simulink model "Vehicle3DOFModelwithLonnLatController"  (R2019b)
settings: Solver=FixedStepAuto  StartTime=0.0  StopTime=150  FixedStep=0.05  RelTol=1e-3
values from neighbouring files (symbols this model uses):
  Ks = 0.1    [Vehicle_Parameters_and_initial_state_comp.m]
  Kv = -10    [Vehicle_Parameters_and_initial_state_comp.m]    (also in sfun_LQRwithFF_YC_2DOF_Vx_changed.m = m/2/L*(lr/Kyf-lf/Kyr))
  m = car.m    [Vehicle_Parameters_and_initial_state_comp.m]    (also in sfun_LQRwithFF_YC_2DOF_Vx_changed.m)
  t_end = 44    [Vehicle_Parameters_and_initial_state_comp.m]
  Ta = 0.1    [Vehicle_Parameters_and_initial_state_comp.m]
  VehPar = [g,m,Iz,lf,lr,l,Kyf,Kyr,mu,FzF,FzR,FxR_max]'    [Vehicle_Parameters_and_initial_state_comp.m]
  VehPos0 = [Tra(1,1);Tra(1,2);Tra(1,3)]    [Vehicle_Parameters_and_initial_state_comp.m]
  VehSt0 = [0;0;Tra(1,6)]    [Vehicle_Parameters_and_initial_state_comp.m]
undefined symbols (not defined in the file or in its folder): Tra
libraries: simulink x2
settings Model: Creator=pc  LastModifiedBy=YC

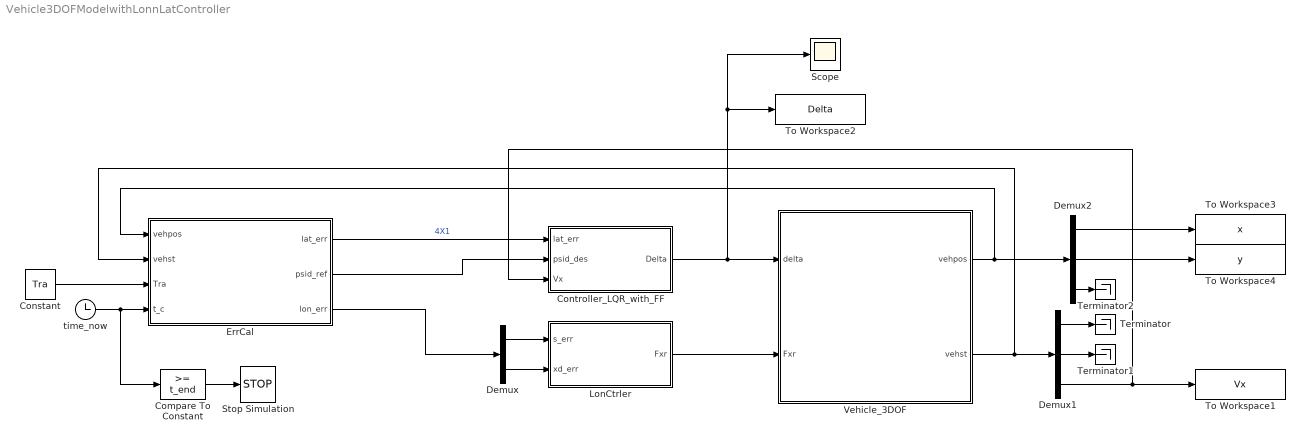
== system Vehicle3DOFModelwithLonnLatController ==
  Compare To Constant : simulink/Logic and Bit Operations/Compare To Constant  relop=>=  const=t_end  OutDataTypeStr=boolean
  Constant : Constant  Value=Tra
  Controller_LQR_with_FF : Subsystem  VariantControl=Controller_mode==1
  Demux : Demux  Outputs=2
  Demux1 : Demux  Outputs=3
  Demux2 : Demux  Outputs=3
  ErrCal : Subsystem  Variant=on
  LonCtrler : Subsystem
  Scope : Scope
  Stop Simulation : Stop
  Terminator : Terminator
  Terminator1 : Terminator
  Terminator2 : Terminator
  To Workspace1 : ToWorkspace  VariableName=Vx  SampleTime=-1
  To Workspace2 : ToWorkspace  VariableName=Delta  SampleTime=-1
  To Workspace3 : ToWorkspace  VariableName=x  SampleTime=-1
  To Workspace4 : ToWorkspace  VariableName=y  SampleTime=-1
  Vehicle_3DOF : Subsystem
  time_now : Clock
  wires:
  Controller_LQR_with_FF/1(Delta) -> To Workspace2/1, Scope/1, Vehicle_3DOF/1(delta)
  ErrCal/1(lat_err) -> Controller_LQR_with_FF/1(lat_err)  "4X1"
  ErrCal/2(psid_ref) -> Controller_LQR_with_FF/2(psid_des)
  LonCtrler/1(Fxr) -> Vehicle_3DOF/2(Fxr)
  Demux/1 -> LonCtrler/1(s_err)
  Demux/2 -> LonCtrler/2(xd_err)
  ErrCal/3(lon_err) -> Demux/1
  Vehicle_3DOF/1(vehpos) -> ErrCal/1(vehpos), Demux2/1
  Vehicle_3DOF/2(vehst) -> ErrCal/2(vehst), Demux1/1
  Constant/1 -> ErrCal/3(Tra)
  time_now/1 -> ErrCal/4(t_c), Compare To Constant/1
  Demux1/1 -> Terminator/1
  Demux1/2 -> Terminator1/1
  Demux1/3 -> To Workspace1/1, Controller_LQR_with_FF/3(Vx)
  Compare To Constant/1 -> Stop Simulation/1
  Demux2/3 -> Terminator2/1
  Demux2/2 -> To Workspace4/1
  Demux2/1 -> To Workspace3/1

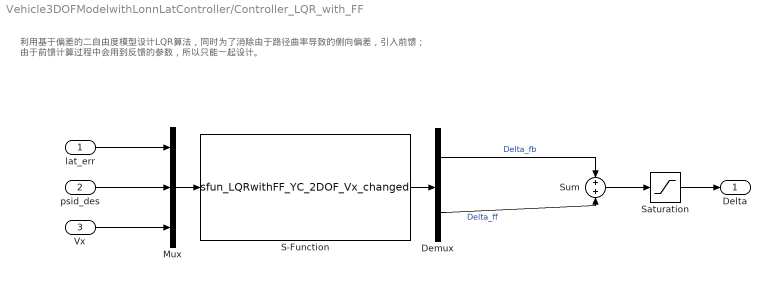
== system Vehicle3DOFModelwithLonnLatController/Controller_LQR_with_FF ==
  note: 利用基于偏差的二自由度模型设计LQR算法，同时为了消除由于路径曲率导致的侧向偏差，引入前馈；
      | 由于前馈计算过程中会用到反馈的参数，所以只能一起设计。
  lat_err : Inport
  psid_des : Inport  Port=2
  Vx : Inport  Port=3
  Demux : Demux  Outputs=2
  Mux : Mux  Inputs=3
  S-Function : S-Function  FunctionName=sfun_LQRwithFF_YC_2DOF_Vx_changed  Parameters=car  SFunctionDeploymentMode=off  EnableBusSupport=off
  Saturation : Saturate  UpperLimit=0.61  LowerLimit=-0.61
  Sum : Sum  Inputs=+|+
  Delta : Outport
  wires:
  Mux/1 -> S-Function/1
  Demux/2 -> Sum/2  "Delta_ff"
  Demux/1 -> Sum/1  "Delta_fb"
  Sum/1 -> Saturation/1
  S-Function/1 -> Demux/1
  lat_err/1 -> Mux/1
  psid_des/1 -> Mux/2
  Vx/1 -> Mux/3
  Saturation/1 -> Delta/1

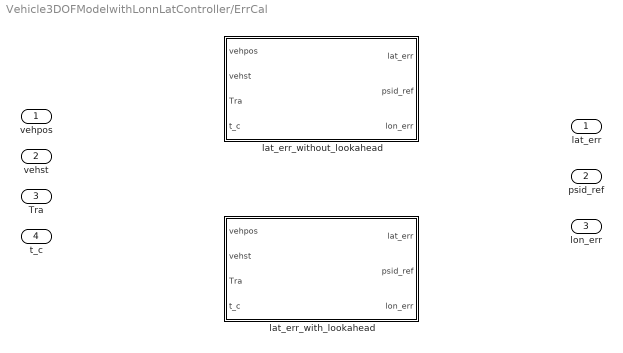
== system Vehicle3DOFModelwithLonnLatController/ErrCal ==
  vehpos : Inport
  vehst : Inport  Port=2
  Tra : Inport  Port=3
  t_c : Inport  Port=4
  lat_err_with_lookahead : Subsystem  VariantControl=Error_Mode==1
  lat_err_without_lookahead : Subsystem  VariantControl=Error_Mode==0
  lat_err : Outport
  psid_ref : Outport  Port=2
  lon_err : Outport  Port=3

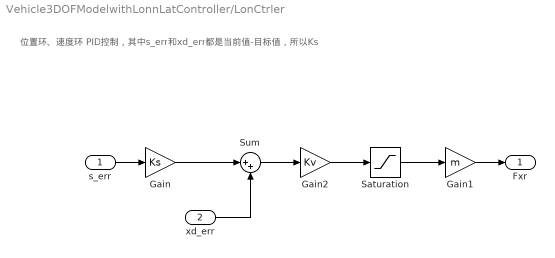
== system Vehicle3DOFModelwithLonnLatController/LonCtrler ==
  note: 位置环、速度环 PID控制，其中s_err和xd_err都是当前值-目标值，所以Ks
  s_err : Inport
  xd_err : Inport  Port=2
  Gain : Gain  Gain=Ks
  Gain1 : Gain  Gain=m
  Gain2 : Gain  Gain=Kv
  Saturation : Saturate  UpperLimit=3  LowerLimit=-3
  Sum : Sum  Inputs=|++
  Fxr : Outport
  wires:
  s_err/1 -> Gain/1
  xd_err/1 -> Sum/2
  Gain/1 -> Sum/1
  Sum/1 -> Gain2/1
  Gain1/1 -> Fxr/1
  Gain2/1 -> Saturation/1
  Saturation/1 -> Gain1/1

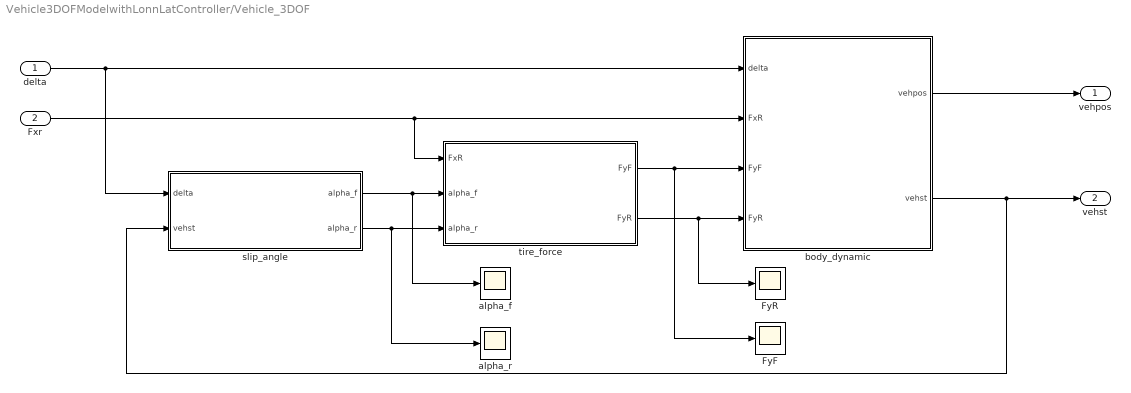
== system Vehicle3DOFModelwithLonnLatController/Vehicle_3DOF ==
  delta : Inport
  Fxr : Inport  Port=2
  FyF : Scope
  FyR : Scope
  alpha_f : Scope
  alpha_r : Scope
  body_dynamic : Subsystem
  slip_angle : Subsystem
  tire_force : Subsystem
  vehpos : Outport
  vehst : Outport  Port=2
  wires:
  body_dynamic/2(vehst) -> vehst/1, slip_angle/2(vehst)
  slip_angle/1(alpha_f) -> alpha_f/1, tire_force/2(alpha_f)
  slip_angle/2(alpha_r) -> alpha_r/1, tire_force/3(alpha_r)
  body_dynamic/1(vehpos) -> vehpos/1
  Fxr/1 -> body_dynamic/2(FxR), tire_force/1(FxR)
  tire_force/2(FyR) -> FyR/1, body_dynamic/4(FyR)
  tire_force/1(FyF) -> FyF/1, body_dynamic/3(FyF)
  delta/1 -> slip_angle/1(delta), body_dynamic/1(delta)

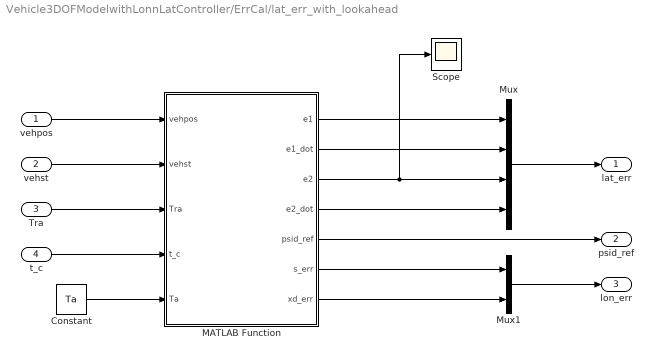
== system Vehicle3DOFModelwithLonnLatController/ErrCal/lat_err_with_lookahead ==
  vehpos : Inport
  vehst : Inport  Port=2
  Tra : Inport  Port=3
  t_c : Inport  Port=4
  Constant : Constant  Value=Ta
  MATLAB Function : MATLAB Function  TreatAsAtomicUnit=on
  Mux : Mux
  Mux1 : Mux  Inputs=2
  Scope : Scope
  lat_err : Outport
  psid_ref : Outport  Port=2
  lon_err : Outport  Port=3
  wires:
  MATLAB Function/2(e1_dot) -> Mux/2
  MATLAB Function/3(e2) -> Scope/1, Mux/3
  Mux/1 -> lat_err/1
  MATLAB Function/1(e1) -> Mux/1
  Tra/1 -> MATLAB Function/3(Tra)
  MATLAB Function/4(e2_dot) -> Mux/4
  MATLAB Function/5(psid_ref) -> psid_ref/1
  vehpos/1 -> MATLAB Function/1(vehpos)
  MATLAB Function/7(xd_err) -> Mux1/2
  MATLAB Function/6(s_err) -> Mux1/1
  Mux1/1 -> lon_err/1
  t_c/1 -> MATLAB Function/4(t_c)
  vehst/1 -> MATLAB Function/2(vehst)
  Constant/1 -> MATLAB Function/5(Ta)

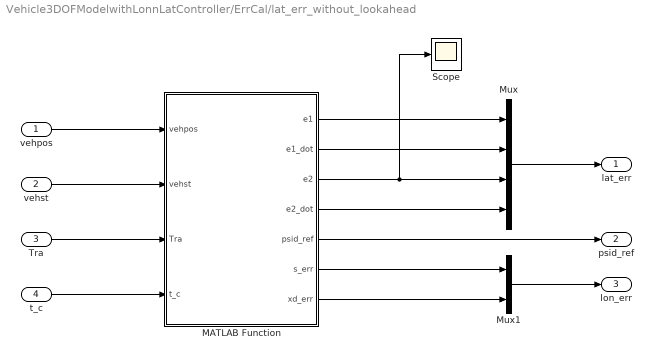
== system Vehicle3DOFModelwithLonnLatController/ErrCal/lat_err_without_lookahead ==
  vehpos : Inport
  vehst : Inport  Port=2
  Tra : Inport  Port=3
  t_c : Inport  Port=4
  MATLAB Function : MATLAB Function  TreatAsAtomicUnit=on
  Mux : Mux
  Mux1 : Mux  Inputs=2
  Scope : Scope
  lat_err : Outport
  psid_ref : Outport  Port=2
  lon_err : Outport  Port=3
  wires:
  MATLAB Function/2(e1_dot) -> Mux/2
  MATLAB Function/3(e2) -> Scope/1, Mux/3
  Mux/1 -> lat_err/1
  MATLAB Function/1(e1) -> Mux/1
  Tra/1 -> MATLAB Function/3(Tra)
  MATLAB Function/4(e2_dot) -> Mux/4
  MATLAB Function/5(psid_ref) -> psid_ref/1
  vehpos/1 -> MATLAB Function/1(vehpos)
  MATLAB Function/7(xd_err) -> Mux1/2
  MATLAB Function/6(s_err) -> Mux1/1
  Mux1/1 -> lon_err/1
  t_c/1 -> MATLAB Function/4(t_c)
  vehst/1 -> MATLAB Function/2(vehst)

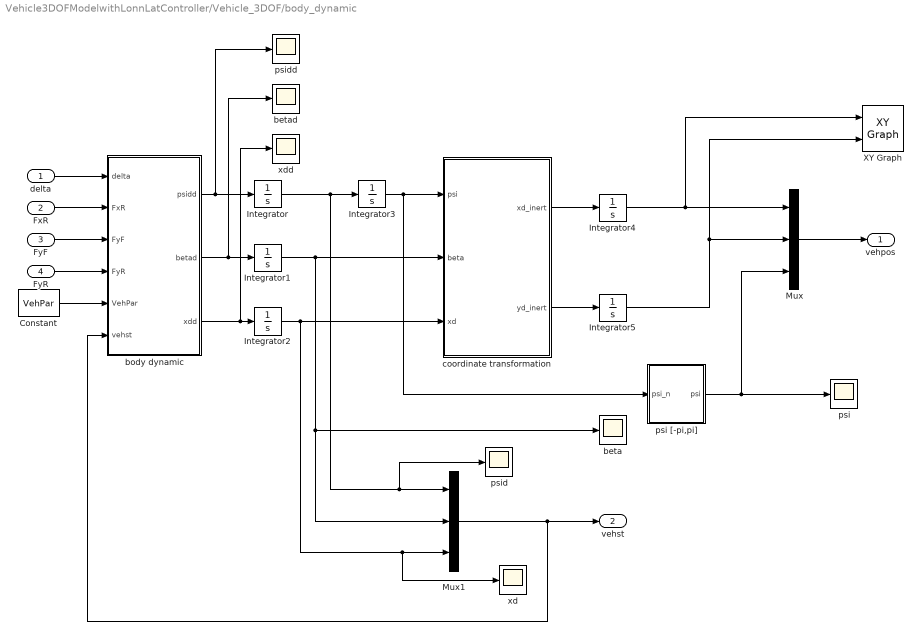
== system Vehicle3DOFModelwithLonnLatController/Vehicle_3DOF/body_dynamic ==
  delta : Inport
  FxR : Inport  Port=2
  FyF : Inport  Port=3
  FyR : Inport  Port=4
  Constant : Constant  Value=VehPar
  Integrator : Integrator  InitialCondition=VehSt0(1)
  Integrator1 : Integrator  InitialCondition=VehSt0(2)
  Integrator2 : Integrator  InitialCondition=VehSt0(3)
  Integrator3 : Integrator  InitialCondition=VehPos0(3)
  Integrator4 : Integrator  InitialCondition=VehPos0(1)
  Integrator5 : Integrator  InitialCondition=VehPos0(2)
  Mux : Mux  Inputs=3
  Mux1 : Mux  Inputs=3
  XY Graph : simulink/Sinks/XY Graph  xmin=-25  xmax=25  ymin=-10  ymax=40  st=-1
  beta : Scope
  betad : Scope
  body dynamic : MATLAB Function  TreatAsAtomicUnit=on
  coordinate transformation : MATLAB Function  TreatAsAtomicUnit=on
  psi : Scope
  psi [-pi,pi] : MATLAB Function  TreatAsAtomicUnit=on
  psid : Scope
  psidd : Scope
  xd : Scope
  xdd : Scope
  vehpos : Outport
  vehst : Outport  Port=2
  wires:
  body dynamic/1(psidd) -> psidd/1, Integrator/1
  body dynamic/3(xdd) -> xdd/1, Integrator2/1
  body dynamic/2(betad) -> Integrator1/1, betad/1
  Constant/1 -> body dynamic/5(VehPar)
  delta/1 -> body dynamic/1(delta)
  FxR/1 -> body dynamic/2(FxR)
  FyF/1 -> body dynamic/3(FyF)
  FyR/1 -> body dynamic/4(FyR)
  Integrator/1 -> Integrator3/1, psid/1, Mux1/1
  Integrator3/1 -> psi [-pi,pi]/1(psi_n), coordinate transformation/1(psi)
  Integrator1/1 -> Mux1/2, beta/1, coordinate transformation/2(beta)
  Integrator2/1 -> Mux1/3, xd/1, coordinate transformation/3(xd)
  coordinate transformation/2(yd_inert) -> Integrator5/1
  coordinate transformation/1(xd_inert) -> Integrator4/1
  Integrator4/1 -> XY Graph/1, Mux/1
  Integrator5/1 -> XY Graph/2, Mux/2
  Mux1/1 -> body dynamic/6(vehst), vehst/1
  Mux/1 -> vehpos/1
  psi [-pi,pi]/1(psi) -> Mux/3, psi/1

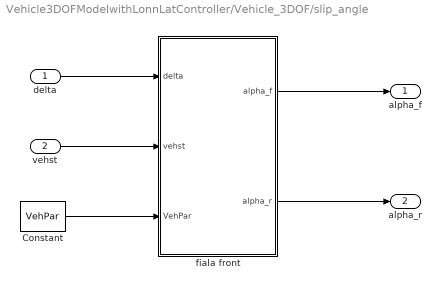
== system Vehicle3DOFModelwithLonnLatController/Vehicle_3DOF/slip_angle ==
  delta : Inport
  vehst : Inport  Port=2
  Constant : Constant  Value=VehPar
  fiala front : MATLAB Function  TreatAsAtomicUnit=on
  alpha_f : Outport
  alpha_r : Outport  Port=2
  wires:
  Constant/1 -> fiala front/3(VehPar)
  delta/1 -> fiala front/1(delta)
  fiala front/1(alpha_f) -> alpha_f/1
  vehst/1 -> fiala front/2(vehst)
  fiala front/2(alpha_r) -> alpha_r/1

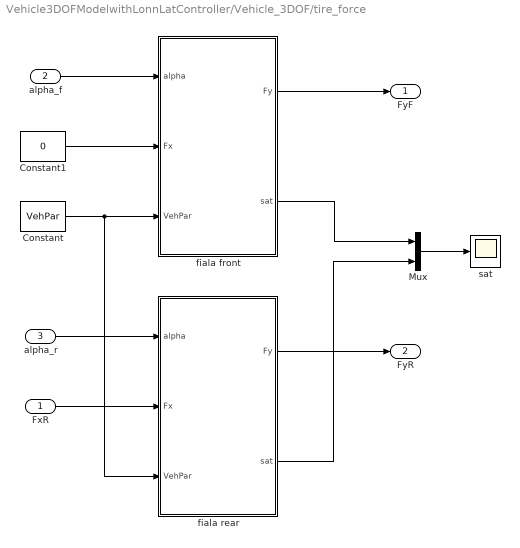
== system Vehicle3DOFModelwithLonnLatController/Vehicle_3DOF/tire_force ==
  FxR : Inport
  alpha_f : Inport  Port=2
  alpha_r : Inport  Port=3
  Constant : Constant  Value=VehPar
  Constant1 : Constant  Value=0
  Mux : Mux  Inputs=2
  fiala front : MATLAB Function  TreatAsAtomicUnit=on
  fiala rear : MATLAB Function  TreatAsAtomicUnit=on
  sat : Scope
  FyF : Outport
  FyR : Outport  Port=2
  wires:
  Constant/1 -> fiala rear/3(VehPar), fiala front/3(VehPar)
  alpha_f/1 -> fiala front/1(alpha)
  FxR/1 -> fiala rear/2(Fx)
  fiala front/1(Fy) -> FyF/1
  Constant1/1 -> fiala front/2(Fx)
  alpha_r/1 -> fiala rear/1(alpha)
  fiala rear/1(Fy) -> FyR/1
  fiala front/2(sat) -> Mux/1
  fiala rear/2(sat) -> Mux/2
  Mux/1 -> sat/1

== matlab function Vehicle3DOFModelwithLonnLatController/ErrCal/lat_err_with_lookahead/MATLAB Function ==
  data: vehpos input; vehst input; Tra input; e1 output; e1_dot output; e2 output; e2_dot output; psid_ref output; s_err output; xd_err output; t_c input; Ta input
function [e1,e1_dot,e2,e2_dot,psid_ref,s_err,xd_err] = fcn(vehpos,vehst,Tra,t_c,Ta)
% % x_ref,y_ref,psi_ref,kappa_ref,n是调试用的，检验这个函数的正确性。已删除

% 车辆实时状态
x_inert=vehpos(1);
y_inert=vehpos(2);
psi=vehpos(3);
Vx=vehst(3);
beta=vehst(2);
psid=vehst(1);
% 规划轨迹
X=Tra(:,1);
Y=Tra(:,2);
PSI=Tra(:,3);
KAPPA=Tra(:,4);
S=Tra(:,5);
V=Tra(:,6);
T=Tra(:,7);

% 寻找距离最近点nearest_point
dX=x_inert-X;
dY=y_inert-Y;
deltaS=sqrt(dX.^2+dY.^2);
[~,n]=min(deltaS);% 索引为n的点即为距离最近点

% 偏差计算，在距离最近点和下一个点的基础上找投影点Matched_Point
tol=0.001;
if abs(X(n+1)-X(n))<tol %直线PnPn+1斜率很大
    x_proj = X(n);
    y_proj = y_inert;
elseif abs(Y(n+1)-Y(n))<tol %直线PnPn+1斜率为零
    x_proj = x_inert;
    y_proj = Y(n);
else
    k1=(Y(n+1)-Y(n))/(X(n+1)-X(n));%直线PnPn+1斜率
    k2=-1/k1;
    x_proj = (y_inert-Y(n)+k1*X(n)-k2*x_inert)/(k1-k2);% 根据两条直线的斜率和点方程求投影点
    y_proj = y_inert+k2*(x_proj-x_inert);
end

dist_p = sqrt((X(n+1)-x_proj)^2+(Y(n+1)-y_proj)^2);
% 在投影点以及参考轨迹的基础上做预瞄，找预瞄参考点
for m=n+1:length(X)-1 % 有超出终点的风险 
    if dist_p-Vx*Ta<0
        dist_p = dist_p+sqrt((X(m+1)-X(m))^2+(Y(m+1)-Y(m))^2);
    else
        break;
    end
end
dist_q = dist_p-Vx*Ta;% 相对m点往回多远距离
dist_r = sqrt((X(m-1)-X(m))^2+(Y(m-1)-Y(m))^2);% m和m-1点之间的距离
ratio1 = dist_q/dist_r;

x_ref = X(m)-ratio1*(X(m)-X(m-1));% 预瞄参考点
y_ref = Y(m)-ratio1*(Y(m)-Y(m-1));
psi_ref = ratio1*PSI(m-1)+(1-ratio1)*PSI(m);
kappa_ref = ratio1*KAPPA(m-1)+(1-ratio1)*KAPPA(m);

% 偏差计算,以参考轨迹坐标系计算偏差,当前点与参考点的差值（当前点-参考点）
e1=(y_inert-y_ref).*cos(psi_ref)-(x_inert-x_ref).*sin(psi_ref);
% e1=(y_inert-y_ref).*cos(psi)-(x_inert-x_ref).*sin(psi);
e2=psi-psi_ref;
if e2<=-pi % 因为psi是(-pi,pi]，是有界的,防止越界时在-pi,pi之间反复越界跳
    e2=2*pi+e2;
elseif e2>pi
    e2=e2-2*pi;
end
e1_dot=Vx.*sin(e2);
% e1_dot=yd+Vx*e2;
e2_dot=psid-Vx.*kappa_ref;
psid_ref=Vx.*kappa_ref;
%预瞄
% e1=e1+Vx*Ta*sin(psid*Ta/2+yd/Vx);% 考虑到车辆的平动和旋转，但是近似的
e1=e1+Vx*Ta*sin(beta); % 仅考虑车辆的平动
e2=e2+psid*Ta; 

% % 纵向参考点以时间来确定
deltaT=abs(t_c-T);
[~,r]=min(deltaT);% 时刻最近点
r0=r(1);% 防止出现在两个时刻正中间
% 求时间吻合的插值点，作为纵向位置的参考点ref Point
t_p=T(r0+1)-t_c;
a_p=(V(r0+1)-V(r0))/(T(r0+1)-T(r0));
s_p=V(r0+1)*t_p-0.5*a_p*t_p^2;%ref Point到时刻最近点的下一点的距离
% 求match Point到ref Point的距离偏差与速度偏差（速度用当前位置的速度），偏差是:当前点-目标点
s_err=(S(n+1)-dist_p)-(S(r0+1)-s_p);
xd_err=Vx-(V(r0+1)-a_p*t_p);
end

== matlab function Vehicle3DOFModelwithLonnLatController/ErrCal/lat_err_without_lookahead/MATLAB Function ==
  data: vehpos input; vehst input; Tra input; e1 output; e1_dot output; e2 output; e2_dot output; psid_ref output; s_err output; xd_err output; t_c input
function [e1,e1_dot,e2,e2_dot,psid_ref,s_err,xd_err] = fcn(vehpos,vehst,Tra,t_c)
% % x_ref,y_ref,psi_ref,kappa_ref,n是调试用的，检验这个函数的正确性。已删除

% 车辆实时状态
x_inert=vehpos(1);
y_inert=vehpos(2);
psi=vehpos(3);
Vx=vehst(3);
psid=vehst(1);
% 规划轨迹
X=Tra(:,1);
Y=Tra(:,2);
PSI=Tra(:,3);
KAPPA=Tra(:,4);
S=Tra(:,5);
V=Tra(:,6);
T=Tra(:,7);

% 寻找距离最近点nearest_point
dX=x_inert-X;
dY=y_inert-Y;
deltaS=sqrt(dX.^2+dY.^2);
[~,n]=min(deltaS);% 索引为n的点即为距离最近点

% 偏差计算，在距离最近点和下一个点的基础上找投影点Matched_Point
tol=0.001;
if abs(X(n+1)-X(n))<tol %直线PnPn+1斜率很大
    x_proj = X(n);
    y_proj = y_inert;
elseif abs(Y(n+1)-Y(n))<tol %直线PnPn+1斜率为零
    x_proj = x_inert;
    y_proj = Y(n);
else
    k1=(Y(n+1)-Y(n))/(X(n+1)-X(n));%直线PnPn+1斜率
    k2=-1/k1;
    x_proj = (y_inert-Y(n)+k1*X(n)-k2*x_inert)/(k1-k2);% 根据两条直线的斜率和点方程求投影点
    y_proj = y_inert+k2*(x_proj-x_inert);
end
% 将投影点作为最终参考点
x_ref = x_proj;
y_ref = y_proj;

dist = sqrt((X(n+1)-X(n))^2+(Y(n+1)-Y(n))^2);
dist_p = sqrt((X(n+1)-x_proj)^2+(Y(n+1)-y_proj)^2);
ratio = dist_p/dist;
psi_ref = ratio*PSI(n)+(1-ratio)*PSI(n+1);
kappa_ref = ratio*KAPPA(n)+(1-ratio)*KAPPA(n+1);

% 偏差计算,以参考轨迹坐标系计算偏差,当前点与参考点的差值（当前点-参考点）
e1=(y_inert-y_ref).*cos(psi_ref)-(x_inert-x_ref).*sin(psi_ref);
% e1=(y_inert-y_ref).*cos(psi)-(x_inert-x_ref).*sin(psi);
e2=psi-psi_ref;
if e2<=-pi % 因为psi是(-pi,pi]，是有界的,防止越界时在-pi,pi之间反复越界跳
    e2=2*pi+e2;
elseif e2>pi
    e2=e2-2*pi;
end
e1_dot=Vx.*sin(e2);
% e1_dot=yd+Vx*e2;
e2_dot=psid-Vx.*kappa_ref;
psid_ref=Vx.*kappa_ref;

% % 纵向参考点以时间来确定
deltaT=abs(t_c-T);
[~,r]=min(deltaT);% 时刻最近点
r0=r(1);% 防止出现在两个时刻正中间
% 求时间吻合的插值点，作为纵向位置的参考点ref Point
t_p=T(r0+1)-t_c;
a_p=(V(r0+1)-V(r0))/(T(r0+1)-T(r0));
s_p=V(r0+1)*t_p-0.5*a_p*t_p^2;%ref Point到时刻最近点的下一点的距离
% 求match Point到ref Point的距离偏差与速度偏差（速度用当前位置的速度），偏差是:当前点-目标点
s_err=(S(n+1)-dist_p)-(S(r0+1)-s_p);
xd_err=Vx-(V(r0+1)-a_p*t_p);
end

== matlab function Vehicle3DOFModelwithLonnLatController/Vehicle_3DOF/body_dynamic/psi [-pi,pi] ==
  data: psi_n input; psi output
function psi = fcn(psi_n)

psi=mod(psi_n,2*pi);
if psi>pi
    psi = psi-2*pi;
end

end

== matlab function Vehicle3DOFModelwithLonnLatController/Vehicle_3DOF/body_dynamic/body dynamic ==
  data: delta input; FxR input; psidd output size=1; FyF input; FyR input; VehPar input; betad output size=1; xdd output size=1; vehst input
function [psidd,betad,xdd] = fcn(delta,FxR,FyF,FyR,VehPar,vehst)
m=VehPar(2);
Iz=VehPar(3);
a=VehPar(4);
b=VehPar(5);

psid=vehst(1);
beta=vehst(2);
xd=vehst(3);

betad = 1/(m*xd)*(FyF + FyR) - psid;         
psidd = 1/Iz*(a*FyF-b*FyR);                   
xdd = 1/m*(FxR-FyF*delta)+psid*xd*beta;  
% xdd = 1/m*(FxR-FyF*sin(delta))+psid*xd*beta;  
end

== matlab function Vehicle3DOFModelwithLonnLatController/Vehicle_3DOF/body_dynamic/coordinate transformation ==
  data: psi input; beta input; xd_inert output; xd input; yd_inert output
function [xd_inert,yd_inert] = fcn(psi,beta,xd)
% coordinate transformation
xd_inert = xd * (cos(psi) - beta * sin(psi));
yd_inert = xd * (sin(psi) + beta * cos(psi));
end

== matlab function Vehicle3DOFModelwithLonnLatController/Vehicle_3DOF/slip_angle/fiala front ==
  data: delta input; vehst input; alpha_f output; VehPar input; alpha_r output
function [alpha_f,alpha_r] = Slip_Angle(delta,vehst,VehPar)
% slip angle

lf = VehPar(4);
lr = VehPar(5);

psid = vehst(1);
beta = vehst(2);
xd = vehst(3);

alpha_f = atan(beta+lf.*psid./xd)-delta;
alpha_r = atan(beta-lr.*psid./xd);
end

== matlab function Vehicle3DOFModelwithLonnLatController/Vehicle_3DOF/tire_force/fiala front ==
  data: alpha input; Fx input; Fy output; VehPar input; sat output
function [Fy,sat]  = fiala_front(alpha,Fx,VehPar)
% fiala tire model

mu = VehPar(9);
Fz = VehPar(10);% 前轮用FzF，后轮用FzR
Ca = VehPar(7);% 前轮用CaF，后轮用CaR

z = tan(alpha);% slip_angle
xi = sqrt((mu*Fz)^2 - Fx^2)/(mu*Fz);% derating factor
tan_alpha_sl = 3*xi*mu*Fz/Ca;
alpha_sl = atan(tan_alpha_sl);% critical slip_angle
% lateral force calculate
if abs(alpha) < alpha_sl
Fy = -Ca*z + Ca^2/(3*xi*mu*Fz)*abs(z).*z - Ca^3/(27*xi^2*mu^2*Fz^2)*z.^3;
sat = 0;
else
Fy = -xi*mu*Fz*sign(alpha);
sat = 1;
end
end

== matlab function Vehicle3DOFModelwithLonnLatController/Vehicle_3DOF/tire_force/fiala rear ==
  data: alpha input; Fx input; Fy output; VehPar input; sat output
function [Fy,sat]  = fiala_rear(alpha,Fx,VehPar)
% fiala tire model

mu = VehPar(9);
Fz = VehPar(11);% 前轮用FzF，后轮用FzR
Ca = VehPar(8);% 前轮用CaF，后轮用CaR

z = tan(alpha);% slip_angle
xi = sqrt((mu*Fz)^2 - Fx^2)/(mu*Fz);% derating factor
tan_alpha_sl = 3*xi*mu*Fz/Ca;
alpha_sl = atan(tan_alpha_sl);% critical slip_angle
% lateral force calculate
if abs(alpha) < alpha_sl
Fy = -Ca*z + Ca^2/(3*xi*mu*Fz)*abs(z).*z - Ca^3/(27*xi^2*mu^2*Fz^2)*z.^3;
sat = 0;
else
Fy = -xi*mu*Fz*sign(alpha);
sat = 1;
end
end
